simulink model "syst1"  (Simulink 7.8)
settings: Solver=ode45  SolverMode=SingleTasking  StartTime=0.0  StopTime=10  RelTol=1e-3
undefined symbols (not defined in the file or in its folder): f, Fsat, L, l, L0, m, M, th0, v0, w0, x0
settings Model: Creator=mino  LastModifiedBy=petersson  ExtModeTrigMode=oneshot  ExtModeArmWhenConnect=off
settings DataIOCC: LimitDataPoints=off
settings OptimizationCC: BlockReduction=off  BooleanDataType=off  InitFltsAndDblsToZero=on
settings DebuggingCC: SaveWithParameterizedLinksMsg=none  SignalResolutionControl=TryResolveAllWithWarning  SolverPrmCheckMsg=none  MultiTaskDSMMsg=warning  MultiTaskCondExecSysMsg=none  FcnCallInpInsideContextMsg=Use local settings  StrictBusMsg=None
settings HardwareCC: TargetUnknown=on
settings RTWCC: IncludeERTFirstTime=on
settings GRTTargetCC: TargetFcnLib=ansi_tfl_tmw.mat

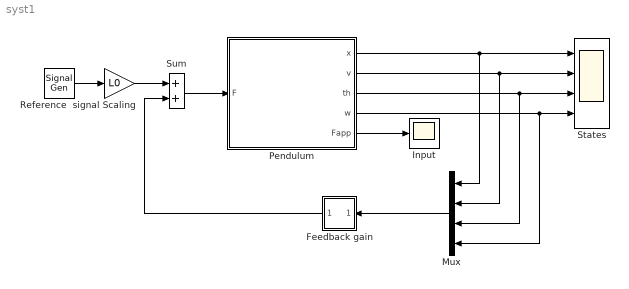
== system syst1 ==
  Feedback gain : Subsystem  mask(Matrix Gain){K=-L}
      mask prompts: K "Gain matrix:"
      mask help: Matrix Gain.
      mask Help: Multiplies input vector by entered matrix to produce output vector (y=Au).
      mask Display: disp('-L')
  Input : Scope
      settings: TickLabels=on  TimeRange=10  YMin=-10  YMax=30  DataFormat=Array
  Mux : Mux
  Pendulum : Subsystem  mask(Pendulum simulated process){x0=[x0 v0 th0 w0], l=l, f=f, m_p=m, M_c=M, Fsat=Fsat, tsample=0.005, sndon=on, inpd=on}
      mask prompts: x0 "Initial cond for the pendulum:"; l "l (length of pendelum)"; f "f (joint friction, pendulum)"; m_p "m (mass of pendulum)"; M_c "M (mass of cart)"; Fsat "Fsat (max. force applied)"; tsample "Sample time for animation:"; sndon "Sound on"; inpd "Display input in animation"
      mask init:
      | g = 9.81; xlimit = 0.5;
      mask Display:
      | text(0.1,0.5,'F')
      | text(0.95,0.95,'x')
      | text(0.95,0.75,'v')
      | text(0.95,0.55,'th')
      | text(0.95,0.35,'w')
      | text(0.87,0.15,'Fapp')
      | plot([0.15 0.65],[0.2 0.2],[0.35 0.35 0.45 0.45],[0.2 0.3 0.3 0.2],[0.4 0.5],[0.3 0.7])
  Reference  signal : SignalGenerator  WaveForm=square  Amplitude=0.3  Frequency=0.1
  Scaling : Gain  Gain=L0  SaturateOnIntegerOverflow=on  OutDataTypeStr=Inherit: Same as input  ParamDataTypeStr=Inherit: Same as input
  States : Scope  NumInputPorts=4
      settings: TimeRange=10  YMin=-0.04~-0.4~0~-10  YMax=0.04~0.4~6~15
  Sum : Sum  SaturateOnIntegerOverflow=on  InputSameDT=on  OutDataTypeStr=Inherit: Same as first input
  wires:
  Pendulum/5(Fapp) -> Input/1
  Feedback gain/1(Out1) -> Sum/2
  Sum/1 -> Pendulum/1(F)
  Scaling/1 -> Sum/1
  Reference  signal/1 -> Scaling/1
  Mux/1 -> Feedback gain/1(In1)
  Pendulum/1(x) -> Mux/1, States/1
  Pendulum/2(v) -> States/2, Mux/2
  Pendulum/3(th) -> States/3, Mux/3
  Pendulum/4(w) -> States/4, Mux/4

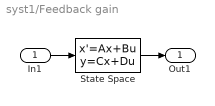
== system syst1/Feedback gain ==
  In1 : Inport
  State Space : StateSpace  A=[]  B=[]  C=[]  D=K
  Out1 : Outport
  wires:
  State Space/1 -> Out1/1
  In1/1 -> State Space/1

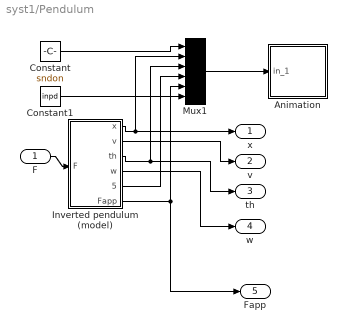
== system syst1/Pendulum ==
  F : Inport
  Animation : Subsystem  mask(Pendulum plot){x0=x0, l=l, xlimit=xlimit, fsat=Fsat, tsample=tsample}
      mask prompts: tsample "ts"
      mask help: Pendulum plot
      mask init:
      | global csv
      | fclose('all');
      | csv = resample(wavread('endp.mat'),1,6);
      mask Help: Pendulum animation function using Handle graphics.
      mask Display: plot([-10 10],[0 0],[-2 -2 2 2],[0 1 1 0],[0 3],[1 5])
  Constant : Constant  Value=sndon
  Constant1 : Constant  Value=inpd
  Inverted pendulum (model) : Subsystem  mask(Pendelum model){x0=x0(1), v0=x0(2), th0=x0(3), w0=x0(4), l=l, f=f, m_p=m_p, M_c=M_c, Fsat=Fsat, xlimit=xlimit}
      mask prompts: m_p "m"; M_c "M"
      mask init:
      | g = 9.81;
  Mux1 : Mux  Inputs=6
  x : Outport  InitialOutput=0
  v : Outport  Port=2  InitialOutput=0
  th : Outport  Port=3  InitialOutput=0
  w : Outport  Port=4  InitialOutput=0
  Fapp : Outport  Port=5  InitialOutput=0
  wires:
  Inverted pendulum (model)/4(w) -> w/1
  Inverted pendulum (model)/2(v) -> v/1
  Inverted pendulum (model)/5(x_stuck) -> Mux1/4
  F/1 -> Inverted pendulum (model)/1(F)
  Constant/1 -> Mux1/1
  Inverted pendulum (model)/1(x) -> x/1, Mux1/2
  Inverted pendulum (model)/3(th) -> th/1, Mux1/3
  Inverted pendulum (model)/6(Fapp) -> Fapp/1, Mux1/5
  Constant1/1 -> Mux1/6
  Mux1/1 -> Animation/1(in_1)

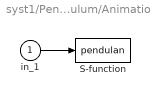
== system syst1/Pendulum/Animation ==
  in_1 : Inport
  S-function : S-Function  FunctionName=pendulan  Parameters="x0; xlimit; l;  fsat; tsample;"  EnableBusSupport=off
      settings: DeleteFcn=pendan([],[],[],'DeleteBlock');
  wires:
  in_1/1 -> S-function/1

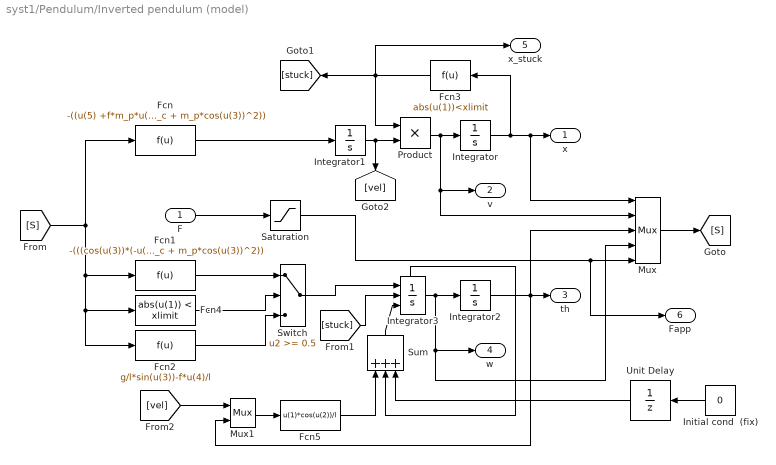
== system syst1/Pendulum/Inverted pendulum (model) ==
  F : Inport
  Fcn : Fcn  Expr=-((u(5) +f*m_p*u(4)*cos(u(3))+ l*m_p*u(4)^2*sin(u(3)) - g*m_p*cos(u(3))*sin(u(3)) - m_p*cos(u(3))*u(2)*u(4)*sin(u(3)))/ (-m_p - M_c + m_p*cos(u(3))^2))
  Fcn1 : Fcn  Expr=-(((cos(u(3))*(-u(5) - l*m_p*u(4)^2*sin(u(3))))/l + ((m_p + M_c)*(-f*u(4)+g*sin(u(3))+ u(2)*u(4)*sin(u(3))))/l)/(-m_p - M_c + m_p*cos(u(3))^2))
  Fcn2 : Fcn  Expr=g/l*sin(u(3))-f*u(4)/l
  Fcn3 : Fcn  Expr=abs(u(1))<xlimit
  Fcn4 : Fcn  Expr=abs(u(1)) < xlimit
  Fcn5 : Fcn  Expr=u(1)*cos(u(2))/l
  Initial cond  (fix) : Constant  Value=0
  Integrator : Integrator  InitialCondition=x0
  Integrator1 : Integrator  InitialCondition=v0
  Integrator2 : Integrator  InitialCondition=th0
  Integrator3 : Integrator  ExternalReset=falling  InitialConditionSource=external  InitialCondition=w0  ShowStatePort=on
  Mux : Mux  Inputs=5
  Mux1 : Mux  Inputs=2
  Product : Product  SaturateOnIntegerOverflow=on  RndMeth=Zero  InputSameDT=on  OutDataTypeStr=Inherit: Same as first input
  Saturation : Saturate  UpperLimit=Fsat  LowerLimit=-Fsat
  Sum : Sum  Inputs=+++  SaturateOnIntegerOverflow=on  InputSameDT=on  OutDataTypeStr=Inherit: Same as first input
  Switch : Switch  Threshold=0.5  SaturateOnIntegerOverflow=on  InputSameDT=on
  Unit Delay : UnitDelay  X0=w0  SampleTime=0.01
  x : Outport
  v : Outport  Port=2
  th : Outport  Port=3
  w : Outport  Port=4
  x_stuck : Outport  Port=5
  Fapp : Outport  Port=6
  wires:
  Saturation/1 -> Fapp/1, Mux/5
  Fcn3/1 -> x_stuck/1, Product/1, [stuck]
  Product/1 -> Mux/2, v/1, Integrator/1
  Mux/1 -> [S]
  Integrator2/1 -> Mux/3, th/1, Mux1/2
  Integrator3/1 -> w/1, Mux/4, Integrator2/1
  Integrator/1 -> Mux/1, x/1, Fcn3/1
  F/1 -> Saturation/1
  Fcn/1 -> Integrator1/1
  [S] -> Fcn/1, Fcn1/1, Fcn4/1, Fcn2/1
  Switch/1 -> Integrator3/1
  Fcn1/1 -> Switch/1
  Fcn4/1 -> Switch/2
  Fcn2/1 -> Switch/3
  [stuck] -> Integrator3/2
  Integrator1/1 -> Product/2, [vel]
  Sum/1 -> Integrator3/3
  Mux1/1 -> Fcn5/1
  [vel] -> Mux1/1
  Fcn5/1 -> Sum/1
  Integrator3/State -> Sum/2
  Unit Delay/1 -> Sum/3
  Initial cond  (fix)/1 -> Unit Delay/1
